simulink model "Template"  (R2025b)
settings: Solver=FixedStepAuto  StartTime=0.0  StopTime=inf  FixedStep=Ts  RelTol=1e-3
model workspace (MATLAB code in the model file):
  | motor_max_torque = 2.2;
  | gear_ratio = [70/16; 40/16; 1];
  | 
  | u_max =   motor_max_torque * gear_ratio;
  | u_min = - motor_max_torque * gear_ratio;
  | 
  | voltage_max    = 15;
  | torque2voltage = voltage_max ./ u_max;
  | 
  | Ts = 1e-3;
  | pp = 14;
undefined symbols (not defined in the file): effort, effort_SL_Info, position, position_SL_Info
libraries: ros2lib x3, eeGeneralControl x1
settings Model: Creator=Asus  LastModifiedBy=Asus
settings OptimizationCC: DefaultParameterBehavior=Inlined  EnhancedBackFolding=on  PassReuseOutputArgsAs=Individual arguments  ZeroExternalMemoryAtStartup=off  ZeroInternalMemoryAtStartup=off  MaxStackSize=64  OptimizeBlockOrder=speed  DifferentSizesBufferReuse=on  OptimizationCustomize=off  EfficientTunableParamExpr=on
settings DebuggingCC: ParameterTunabilityLossMsg=error
settings SFSimCC: MATLABDynamicMemAlloc=off
settings RTWCC: SystemTargetFile=ert.tlc  HardwareBoard=Robot Operating System 2 (ROS 2)  TLCOptions="-aInlineSetEventsForThisBaseRateFcn=TLC_FALSE -aSuppressMultiTaskScheduler=TLC_FALSE  -aRateBasedStepFcn=0"  TemplateMakefile=ert_default_tmf  Toolchain=Colcon Tools  TargetLang=C++  Description=Embedded Coder
settings CodeAppCC: ForceParamTrailComments=on  IgnoreCustomStorageClasses=off  MaxIdLength=95.0  OperatorAnnotations=on  SimulinkDataObjDesc=on  SFDataObjDesc=on  InsertBlockDesc=on
settings ERTTargetCC: RootIOFormat=Structure reference  CodeInterfacePackaging=C++ class

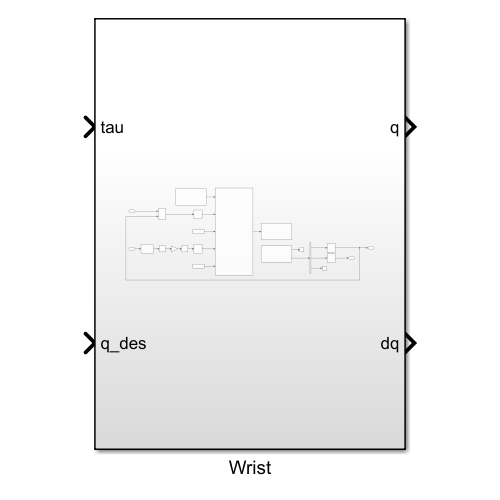
[thumbnail: Simulink's stored preview of the top-level diagram]
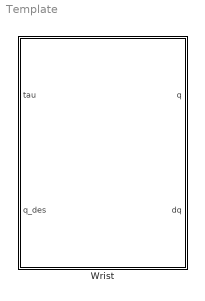
== system Template ==
  Wrist : Subsystem

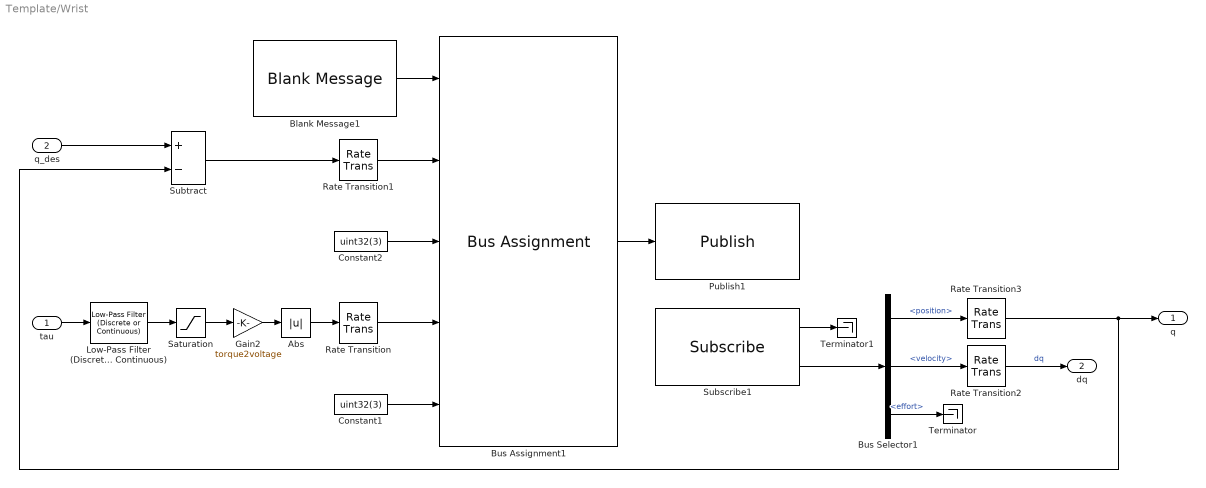
== system Template/Wrist ==
  tau : Inport
  q_des : Inport  Port=2
  Abs : Abs  SaturateOnIntegerOverflow=off
  Blank Message1 : ros2lib/Blank Message  messageClass=Message  entityType=sensor_msgs/JointState  messageType=sensor_msgs/JointState  SampleTime=0.02
  Bus Assignment1 : BusAssignment  AssignedSignals=position,position_SL_Info.CurrentLength,effort,effort_SL_Info.CurrentLength
  Bus Selector1 : BusSelector  OutputSignals=position,velocity,effort
  Constant1 : Constant  Value=uint32(3)
  Constant2 : Constant  Value=uint32(3)
  Gain2 : Gain  Gain=torque2voltage
  Low-Pass Filter (Discrete or Continuous) : eeGeneralControl/Low-Pass Filter (Discrete or Continuous)  K=1  T=0.001  B=inf  A=-inf  init_option=Inherited from block input  x0=0  Ts=-1
  Publish1 : ros2lib/Publish  topicSource=Specify your own  topic=/joint_desireds  messageType=sensor_msgs/JointState  QOSHistory=Keep last  QOSDepth=10  QOSReliability=Reliable  QOSDurability=Volatile  QOSDeadline=Inf  QOSLifespan=Inf  QOSLiveliness=Automatic  QOSLeaseDuration=Inf  QOSAvoidROSNamespaceConventions=off
  Rate Transition : RateTransition  OutPortSampleTime=0.02
  Rate Transition1 : RateTransition  OutPortSampleTime=0.02
  Rate Transition2 : RateTransition  OutPortSampleTime=Ts
  Rate Transition3 : RateTransition  OutPortSampleTime=Ts
  Saturation : Saturate  UpperLimit=u_max  LowerLimit=u_min
  Subscribe1 : ros2lib/Subscribe  topicSource=Select from ROS network  topic=/joint_states  messageType=sensor_msgs/JointState  sampleTime=0.02  QOSHistory=Keep all  QOSDepth=3  QOSReliability=Best effort  QOSDurability=Volatile  QOSDeadline=Inf  QOSLifespan=Inf  QOSLiveliness=Automatic  QOSLeaseDuration=Inf  QOSAvoidROSNamespaceConventions=off
  Subtract : Sum  Inputs=+-
  Terminator : Terminator
  Terminator1 : Terminator
  q : Outport
  dq : Outport  Port=2
  wires:
  Rate Transition1/1 -> Bus Assignment1/2
  Bus Selector1/3 -> Terminator/1  "<effort>"
  Bus Selector1/1 -> Rate Transition3/1  "<position>"
  Rate Transition2/1 -> dq/1  "dq"
  Constant1/1 -> Bus Assignment1/5
  Subscribe1/2 -> Bus Selector1/1
  Rate Transition3/1 -> Subtract/2, q/1
  Blank Message1/1 -> Bus Assignment1/1
  Bus Selector1/2 -> Rate Transition2/1  "<velocity>"
  Constant2/1 -> Bus Assignment1/3
  Abs/1 -> Rate Transition/1
  Subscribe1/1 -> Terminator1/1
  Bus Assignment1/1 -> Publish1/1
  Gain2/1 -> Abs/1
  Rate Transition/1 -> Bus Assignment1/4
  Saturation/1 -> Gain2/1
  Subtract/1 -> Rate Transition1/1
  q_des/1 -> Subtract/1
  Low-Pass Filter (Discrete or Continuous)/1 -> Saturation/1
  tau/1 -> Low-Pass Filter (Discrete or Continuous)/1
